simulink model "lab6"  (R2018b)
settings: Solver=FixedStepDiscrete  StartTime=0.0  StopTime=6.5  FixedStep=0.01  RelTol=1e-3
undefined symbols (not defined in the file): DiscIntNeverNeededParam, lab3_demo_fun
settings Model: Creator=user  LastModifiedBy=user

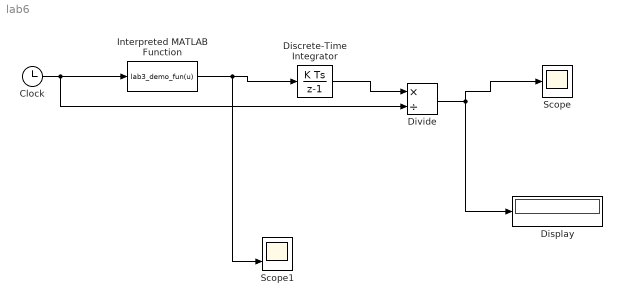
== system lab6 ==
  Clock : Clock
  Discrete-Time Integrator : DiscreteIntegrator  SampleTime=-1  ICPrevOutput=DiscIntNeverNeededParam  ICPrevScaledInput=DiscIntNeverNeededParam
  Display : Display
  Divide : Product  Inputs=*/
  Interpreted MATLAB Function : MATLABFcn  MATLABFcn=lab3_demo_fun(u)
  Scope : Scope
  Scope1 : Scope  NumInputPorts=2
  wires:
  Clock/1 -> Divide/2, Interpreted MATLAB Function/1
  Interpreted MATLAB Function/1 -> Scope1/2, Discrete-Time Integrator/1
  Discrete-Time Integrator/1 -> Divide/1
  Divide/1 -> Scope/1, Display/1
